simulink model "Traj_track_Mechanum_robot_Exp"  (R2024b)
settings: Solver=ode4  StartTime=0.0  StopTime=100  FixedStep=0.02  RelTol=1e-3  EnableMultiTasking=on
libraries: arduinolib x20, slpidlib x8
settings Model: ExtModeTrigDuration=2  Creator=my  LastModifiedBy=my
settings SolverCC: AutoInsertRateTranBlk=on
settings DataIOCC: SaveOutput=off  SignalLogging=off  DSMLogging=off  SaveTime=off  ReturnWorkspaceOutputs=off
settings OptimizationCC: EnhancedBackFolding=on  PassReuseOutputArgsAs=Individual arguments  ZeroExternalMemoryAtStartup=off  ZeroInternalMemoryAtStartup=off  MaxStackSize=64  OptimizeBlockOrder=speed  DifferentSizesBufferReuse=on  OptimizationCustomize=off  EfficientTunableParamExpr=on
settings DebuggingCC: ParameterTunabilityLossMsg=error
settings HardwareCC: ProdBitPerInt=16  ProdBitPerPointer=16  ProdBitPerSizeT=16  ProdBitPerPtrDiffT=16  ProdLargestAtomicFloat=None  ProdWordSize=8  ProdHWDeviceType=Atmel->AVR  UseEmbeddedCoderFeatures=off  UseSimulinkCoderFeatures=off
settings SFSimCC: MATLABDynamicMemAlloc=off
settings RTWCC: Description=Embedded Coder  SystemTargetFile=ert.tlc  HardwareBoard=Arduino Mega 2560  TemplateMakefile=ert_default_tmf  Toolchain=Arduino AVR  BuildConfiguration=Faster Runs
settings CodeAppCC: ForceParamTrailComments=on  IgnoreCustomStorageClasses=off  OperatorAnnotations=on  SimulinkDataObjDesc=on  SFDataObjDesc=on  MangleLength=10  InsertBlockDesc=on
settings ERTTargetCC: SupportContinuousTime=on  SupportNonInlinedSFcns=on  SupportVariableSizeSignals=on  ExtModeTransport=3  ExtModeStaticAlloc=on  ExtModeAutomaticAllocSize=off  ExtModeStaticAllocSize=2048  ExtModeMexFile=ext_xcp  ExtModeIntrfLevel=Level2 - Open  InlinedParameterPlacement=Hierarchical

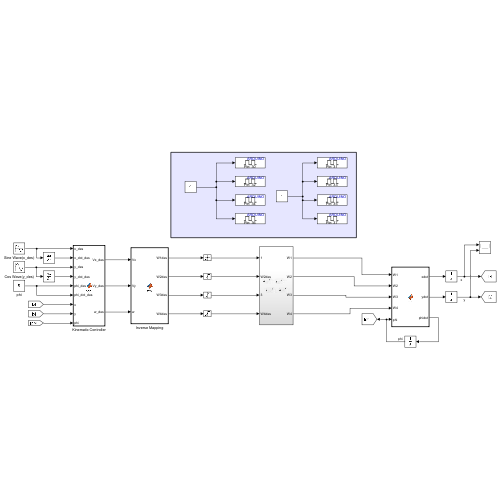
[thumbnail: Simulink's stored preview of the top-level diagram]
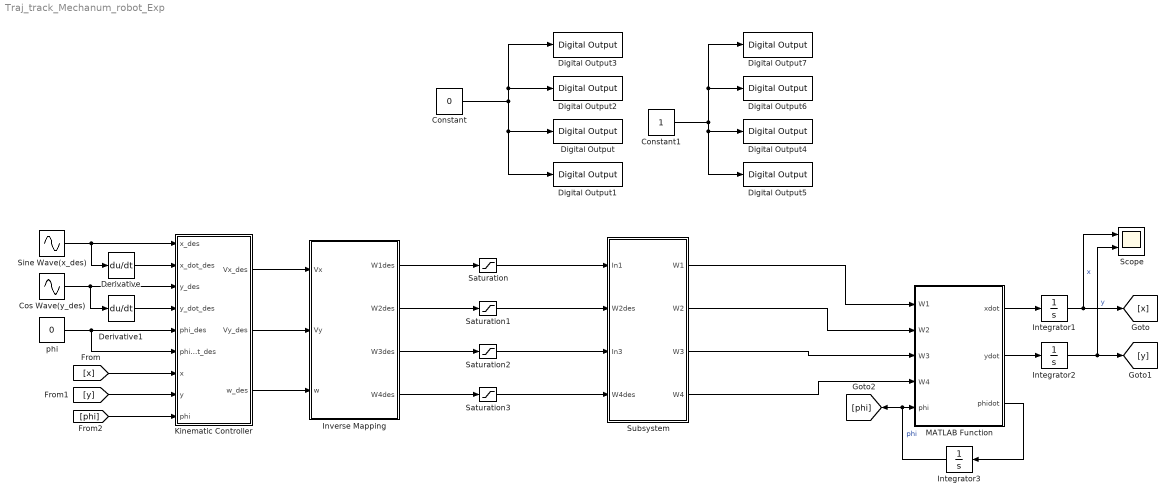
== system Traj_track_Mechanum_robot_Exp ==
  Constant : Constant  Value=0
  Constant1 : Constant
  Cos Wave(y_des) : Sin  Frequency=0.1  Phase=pi/2  SampleTime=0
  Derivative : Derivative
  Derivative1 : Derivative
  Digital Output : arduinolib/Digital Output  pinNumber=34  Direction=output  blockPlatform=arduino
  Digital Output1 : arduinolib/Digital Output  pinNumber=36  Direction=output  blockPlatform=arduino
  Digital Output2 : arduinolib/Digital Output  pinNumber=32  Direction=output  blockPlatform=arduino
  Digital Output3 : arduinolib/Digital Output  pinNumber=30  Direction=output  blockPlatform=arduino
  Digital Output4 : arduinolib/Digital Output  pinNumber=35  Direction=output  blockPlatform=arduino
  Digital Output5 : arduinolib/Digital Output  pinNumber=37  Direction=output  blockPlatform=arduino
  Digital Output6 : arduinolib/Digital Output  pinNumber=33  Direction=output  blockPlatform=arduino
  Digital Output7 : arduinolib/Digital Output  pinNumber=31  Direction=output  blockPlatform=arduino
  Integrator1 : Integrator
  Integrator2 : Integrator
  Integrator3 : Integrator
  Inverse Mapping : MATLAB Function  TreatAsAtomicUnit=on
  Kinematic Controller : MATLAB Function  TreatAsAtomicUnit=on
  MATLAB Function : MATLAB Function  TreatAsAtomicUnit=on
  Saturation : Saturate  UpperLimit=300  LowerLimit=-300
  Saturation1 : Saturate  UpperLimit=117  LowerLimit=-117
  Saturation2 : Saturate  UpperLimit=117  LowerLimit=-117
  Saturation3 : Saturate  UpperLimit=117  LowerLimit=-117
  Scope : Scope  NumInputPorts=2
  Sine Wave(x_des) : Sin  Frequency=0.1  SampleTime=0
  Subsystem : Subsystem
  phi : Constant  Value=0
  wires:
  Constant/1 -> Digital Output1/1, Digital Output/1, Digital Output2/1, Digital Output3/1
  Constant1/1 -> Digital Output6/1, Digital Output7/1, Digital Output5/1, Digital Output4/1
  Integrator2/1 -> Scope/2, [y]  "y"
  MATLAB Function/2(ydot) -> Integrator2/1
  MATLAB Function/1(xdot) -> Integrator1/1
  Integrator3/1 -> [phi], MATLAB Function/5(phi)  "phi"
  MATLAB Function/3(phidot) -> Integrator3/1
  Integrator1/1 -> Scope/1, [x]  "x"
  Saturation/1 -> Subsystem/1(In1)
  Saturation1/1 -> Subsystem/2(W2des)
  Saturation2/1 -> Subsystem/3(In3)
  Saturation3/1 -> Subsystem/4(W4des)
  Subsystem/1(W1) -> MATLAB Function/1(W1)
  Subsystem/2(W2) -> MATLAB Function/2(W2)
  Subsystem/3(W3) -> MATLAB Function/3(W3)
  Subsystem/4(W4) -> MATLAB Function/4(W4)
  Cos Wave(y_des)/1 -> Derivative1/1, Kinematic Controller/3(y_des)
  [phi] -> Kinematic Controller/9(phi)
  Inverse Mapping/1(W1des) -> Saturation/1
  Inverse Mapping/4(W4des) -> Saturation3/1
  [x] -> Kinematic Controller/7(x)
  Derivative/1 -> Kinematic Controller/2(x_dot_des)
  Kinematic Controller/1(Vx_des) -> Inverse Mapping/1(Vx)
  Kinematic Controller/2(Vy_des) -> Inverse Mapping/2(Vy)
  Inverse Mapping/3(W3des) -> Saturation2/1
  Kinematic Controller/3(w_des) -> Inverse Mapping/3(w)
  [y] -> Kinematic Controller/8(y)
  Inverse Mapping/2(W2des) -> Saturation1/1
  Sine Wave(x_des)/1 -> Derivative/1, Kinematic Controller/1(x_des)
  Derivative1/1 -> Kinematic Controller/4(y_dot_des)
  phi/1 -> Kinematic Controller/6(phi_dot_des), Kinematic Controller/5(phi_des)

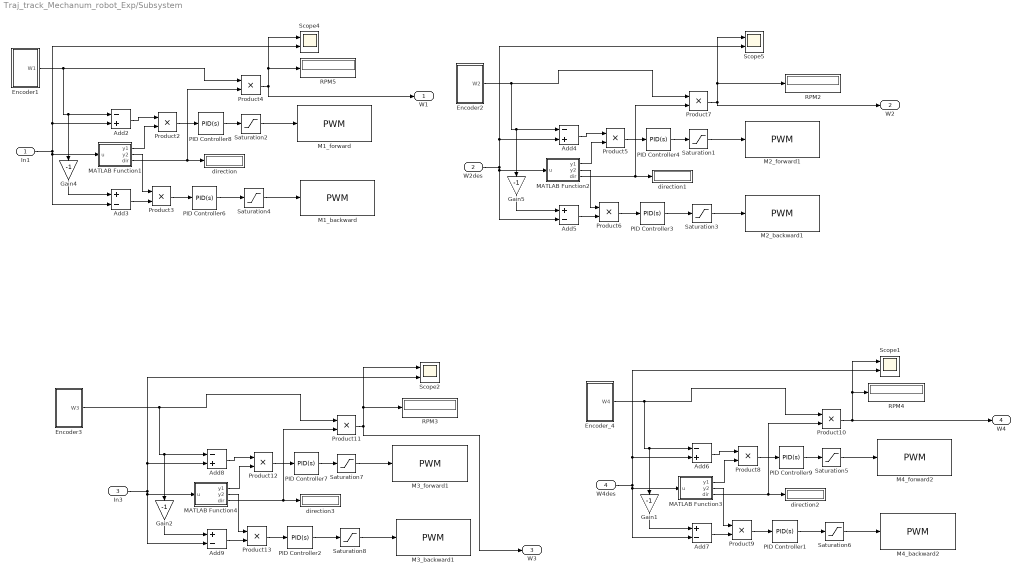
== system Traj_track_Mechanum_robot_Exp/Subsystem ==
  In1 : Inport
  W2des : Inport  Port=2
  In3 : Inport  Port=3
  W4des : Inport  Port=4
  Add{2,4,6,8} (4 alike) : Sum  Inputs=-+
  Add{3,5,7,9} (4 alike) : Sum  Inputs=+-
  Encoder1 : Subsystem
  Encoder2 : Subsystem
  Encoder3 : Subsystem
  Encoder_4 : Subsystem
  Gain{1..2,4..5} (4 alike) : Gain  Gain=-1
  M1_backward : arduinolib/PWM  pinNumber=5  frequencyType=Default  desiredFrequency=490.2  achievableFrequency=490.2
  M1_forward : arduinolib/PWM  pinNumber=4  frequencyType=Default  desiredFrequency=490.2  achievableFrequency=490.2
  M2_backward1 : arduinolib/PWM  pinNumber=7  frequencyType=Default  desiredFrequency=490.2  achievableFrequency=490.2
  M2_forward1 : arduinolib/PWM  pinNumber=6  frequencyType=Default  desiredFrequency=490.2  achievableFrequency=490.2
  M3_backward1 : arduinolib/PWM  pinNumber=10  frequencyType=Default  desiredFrequency=490.2  achievableFrequency=490.2
  M3_forward1 : arduinolib/PWM  pinNumber=9  frequencyType=Default  desiredFrequency=490.2  achievableFrequency=490.2
  M4_backward2 : arduinolib/PWM  pinNumber=12  frequencyType=Default  desiredFrequency=490.2  achievableFrequency=490.2
  M4_forward2 : arduinolib/PWM  pinNumber=11  frequencyType=Default  desiredFrequency=490.2  achievableFrequency=490.2
  MATLAB Function1 : MATLAB Function  TreatAsAtomicUnit=on
  MATLAB Function2 : MATLAB Function  TreatAsAtomicUnit=on
  MATLAB Function3 : MATLAB Function  TreatAsAtomicUnit=on
  MATLAB Function4 : MATLAB Function  TreatAsAtomicUnit=on
  PID Controller{1..4,6..9} (8 alike) : slpidlib/PID Controller  Controller=PID  Form=Parallel  TimeDomain=Continuous-time  UseExternalTs=off  SampleTime=-1  IntegratorMethod=Forward Euler  FilterMethod=Forward Euler  ControllerParametersSource=internal  P=10  I=0  UseKiTs=off  D=0  UseExternalDerivativeSource=off  N=100  UseFilter=on  TunerSelectOption=Transfer Function Based (PID Tuner App)  InitialConditionSource=internal  InitialConditionForIntegrator=0  InitialConditionForFilter=0  DifferentiatorICPrevScaledInput=0  ExternalReset=none  TrackingMode=off  Kt=1  LimitOutput=on  SatLimitsSource=internal  UpperSaturationLimit=255  LowerSaturationLimit=0  LinearizeAsGain=on  AntiWindupMode=none  Kb=1  LimitIntegrator=off  UpperIntegratorSaturationLimit=inf  LowerIntegratorSaturationLimit=-inf  POutMin=[]  POutMax=[]  IOutMin=[]  IOutMax=[]  DOutMin=[]  DOutMax=[]  NOutMin=[]  NOutMax=[]  SumOutMin=[]  SumOutMax=[]  SaturationOutMin=[]  SaturationOutMax=[]  PParamMin=[]  PParamMax=[]  IParamMin=[]  IParamMax=[]  DParamMin=[]  DParamMax=[]  NParamMin=[]  NParamMax=[]  KbParamMin=[]  KbParamMax=[]  KtParamMin=[]  KtParamMax=[]  KbOutMin=[]  KbOutMax=[]  KtOutMin=[]  KtOutMax=[]  IntegratorOutMin=[]  IntegratorOutMax=[]  FilterOutMin=[]  FilterOutMax=[]  SumI1OutMin=[]  SumI1OutMax=[]  SumI2OutMin=[]  SumI2OutMax=[]  SumI3OutMin=[]  SumI3OutMax=[]  SumI4OutMin=[]  SumI4OutMax=[]  SumDOutMin=[]  SumDOutMax=[]  DifferentiatorOutMin=[]  DifferentiatorOutMax=[]  FilterDiffOutCoefMin=[]  FilterDiffOutCoefMax=[]  ReciprocalOutMin=[]  ReciprocalOutMax=[]  SumDenOutMin=[]  SumDenOutMax=[]  SumNumOutMin=[]  SumNumOutMax=[]  DivideOutMin=[]  DivideOutMax=[]  UdiffTsProdOutMin=[]  UdiffTsProdOutMax=[]  NTsProdOutMin=[]  NTsProdOutMax=[]  UintegralTsProdOutMin=[]  UintegralTsProdOutMax=[]  UngainTsProdOutMin=[]  UngainTsProdOutMax=[]  ClampingZeroOutDataTypeStr=Inherit: Inherit via back propagation  ClampingZeroOutMin=[]  ClampingZeroOutMax=[]  FilterDenConstantOutDataTypeStr=Inherit: Inherit via back propagation  FilterDenConstantOutMin=[]  FilterDenConstantOutMax=[]  PCopyOutDataTypeStr=Inherit: Inherit via back propagation  PCopyOutMin=[]  PCopyOutMax=[]  NCopyOutDataTypeStr=Inherit: Inherit via back propagation  NCopyOutMin=[]  NCopyOutMax=[]  IntegratorContinuousStateAttributes=''  IntegratorStateMustResolveToSignalObject=off  IntegratorRTWStateStorageClass=Auto  FilterContinuousStateAttributes=''  FilterStateMustResolveToSignalObject=off  FilterRTWStateStorageClass=Auto  ParallelPVariant=InternalParameters  IdealPVariant=Disabled  IVariant=InternalParameters  DVariant=InternalParameters  IntegratorVariant=Continuous  SatVariant=Enabled  AWVariant=Passthrough  PCopyVariant=Disabled  TRVariant=Disabled  FdbkBlocksVariant=Forward  IdealPFdbkVariant=Disabled  SatFdbkVariant=Disabled  DerivativeFilterVariant=ContFilter  NVariant=InternalParameters  NCopyVariant=Disabled  FilterICVariant=InternalICsFilter  IntegratorICVariant=InternalICs  ExternalResetVariant=Disabled  TRSumVariant=Passthrough  SumFdbkVariant=Disabled  SumVariant=Sum_PID  TsampFilterVariant=InternalTs  TsampNgainVariant=Passthrough  TsampIntegralVariant=Disabled_SignalSpec  ExternalSaturationOutDataTypeStr=Inherit: Same as second input  DerivativeSourceVariant=ErrorSignal  PreIntVariant=InternalPreInt
  Product{2..13} (12 alike) : Product
  RPM{2..5} (4 alike) : Display
  Saturation{1..8} (8 alike) : Saturate  UpperLimit=250  LowerLimit=0
  Scope{1..2,4..5} (4 alike) : Scope  NumInputPorts=2
  direction{,1..3} (4 alike) : Display
  W1 : Outport
  W2 : Outport  Port=2
  W3 : Outport  Port=3
  W4 : Outport  Port=4
  wires:
  MATLAB Function1/2(y2) -> Product3/1
  MATLAB Function1/3(dir) -> Product4/2, direction/1
  In1/1 -> Scope4/2, Add2/2, Add3/2, MATLAB Function1/1(u)
  PID Controller6/1 -> Saturation4/1
  Saturation2/1 -> M1_forward/1
  PID Controller8/1 -> Saturation2/1
  Saturation4/1 -> M1_backward/1
  Add2/1 -> Product2/1
  Encoder1/1(W1) -> Product4/1, Add2/1, Gain4/1
  MATLAB Function1/1(y1) -> Product2/2
  Product2/1 -> PID Controller8/1
  Gain4/1 -> Add3/1
  Product3/1 -> PID Controller6/1
  Add3/1 -> Product3/2
  Add5/1 -> Product6/2
  Product6/1 -> PID Controller3/1
  Gain5/1 -> Add5/1
  Product5/1 -> PID Controller4/1
  MATLAB Function2/1(y1) -> Product5/2
  Encoder2/1(W2) -> Gain5/1, Add4/1, Product7/1
  Add4/1 -> Product5/1
  Saturation3/1 -> M2_backward1/1
  PID Controller4/1 -> Saturation1/1
  Saturation1/1 -> M2_forward1/1
  PID Controller3/1 -> Saturation3/1
  W2des/1 -> MATLAB Function2/1(u), Add5/2, Add4/2, Scope5/2
  MATLAB Function2/3(dir) -> direction1/1, Product7/2
  MATLAB Function2/2(y2) -> Product6/1
  MATLAB Function3/2(y2) -> Product9/1
  MATLAB Function3/3(dir) -> Product10/2, direction2/1
  W4des/1 -> Scope1/2, Add6/2, Add7/2, MATLAB Function3/1(u)
  PID Controller1/1 -> Saturation6/1
  Saturation5/1 -> M4_forward2/1
  PID Controller9/1 -> Saturation5/1
  Saturation6/1 -> M4_backward2/1
  Add6/1 -> Product8/1
  Encoder_4/1(W4) -> Product10/1, Add6/1, Gain1/1
  MATLAB Function3/1(y1) -> Product8/2
  Product8/1 -> PID Controller9/1
  Gain1/1 -> Add7/1
  Product9/1 -> PID Controller1/1
  Add7/1 -> Product9/2
  Product11/1 -> Scope2/1, RPM3/1, W3/1
  Add9/1 -> Product13/2
  Product13/1 -> PID Controller2/1
  Gain2/1 -> Add9/1
  Product12/1 -> PID Controller7/1
  MATLAB Function4/1(y1) -> Product12/2
  Encoder3/1(W3) -> Gain2/1, Add8/1, Product11/1
  Add8/1 -> Product12/1
  Saturation8/1 -> M3_backward1/1
  PID Controller7/1 -> Saturation7/1
  PID Controller2/1 -> Saturation8/1
  In3/1 -> MATLAB Function4/1(u), Add9/2, Add8/2, Scope2/2
  MATLAB Function4/3(dir) -> direction3/1, Product11/2
  MATLAB Function4/2(y2) -> Product13/1
  Saturation7/1 -> M3_forward1/1
  Product10/1 -> RPM4/1, Scope1/1, W4/1
  Product7/1 -> RPM2/1, Scope5/1, W2/1
  Product4/1 -> RPM5/1, Scope4/1, W1/1

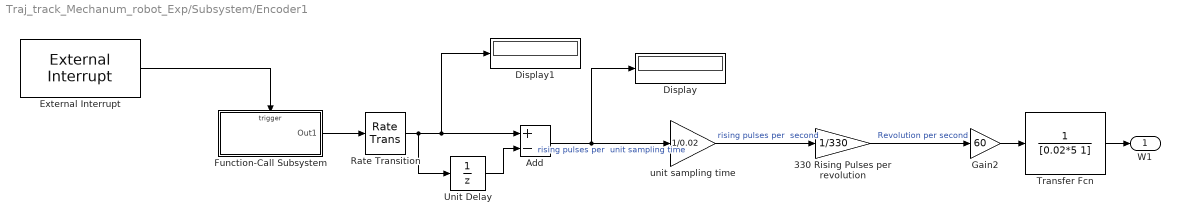
== system Traj_track_Mechanum_robot_Exp/Subsystem/Encoder1 ==
  330 Rising Pulses per revolution : Gain  Gain=1/330
  Add : Sum  Inputs=+-
  Display : Display
  Display1 : Display
  External Interrupt : arduinolib/External Interrupt  Pin=21  PullUp=off  Mode=RISING  InterruptSimulationInput=off
  Function-Call Subsystem : Subsystem  TreatAsAtomicUnit=on
  Gain2 : Gain  Gain=60
  Rate Transition : RateTransition  Integrity=off  Deterministic=off  OutPortSampleTimeOpt=Inherit
  Transfer Fcn : TransferFcn  Denominator=[0.02*5 1]
  Unit Delay : UnitDelay  SampleTime=0.02  HasFrameUpgradeWarning=on
  unit sampling time : Gain  Gain=1/0.02
  W1 : Outport
  wires:
  Transfer Fcn/1 -> W1/1
  Add/1 -> unit sampling time/1, Display/1  "rising pulses per  unit sampling time"
  External Interrupt/1 -> Function-Call Subsystem/Trigger
  Function-Call Subsystem/1(Out1) -> Rate Transition/1
  Gain2/1 -> Transfer Fcn/1
  330 Rising Pulses per revolution/1 -> Gain2/1  "Revolution per second"
  Rate Transition/1 -> Add/1, Display1/1, Unit Delay/1
  unit sampling time/1 -> 330 Rising Pulses per revolution/1  "rising pulses per  second"
  Unit Delay/1 -> Add/2

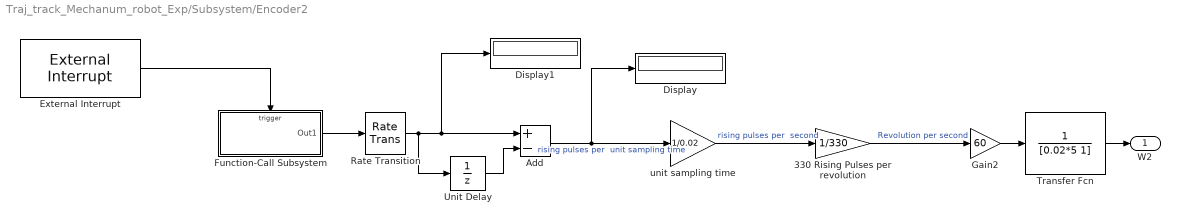
== system Traj_track_Mechanum_robot_Exp/Subsystem/Encoder2 ==
  330 Rising Pulses per revolution : Gain  Gain=1/330
  Add : Sum  Inputs=+-
  Display : Display
  Display1 : Display
  External Interrupt : arduinolib/External Interrupt  Pin=20  PullUp=off  Mode=RISING  InterruptSimulationInput=off
  Function-Call Subsystem : Subsystem  TreatAsAtomicUnit=on
  Gain2 : Gain  Gain=60
  Rate Transition : RateTransition  Integrity=off  Deterministic=off  OutPortSampleTimeOpt=Inherit
  Transfer Fcn : TransferFcn  Denominator=[0.02*5 1]
  Unit Delay : UnitDelay  SampleTime=0.02  HasFrameUpgradeWarning=on
  unit sampling time : Gain  Gain=1/0.02
  W2 : Outport
  wires:
  Unit Delay/1 -> Add/2
  unit sampling time/1 -> 330 Rising Pulses per revolution/1  "rising pulses per  second"
  Rate Transition/1 -> Unit Delay/1, Display1/1, Add/1
  330 Rising Pulses per revolution/1 -> Gain2/1  "Revolution per second"
  Gain2/1 -> Transfer Fcn/1
  Function-Call Subsystem/1(Out1) -> Rate Transition/1
  External Interrupt/1 -> Function-Call Subsystem/Trigger
  Add/1 -> Display/1, unit sampling time/1  "rising pulses per  unit sampling time"
  Transfer Fcn/1 -> W2/1

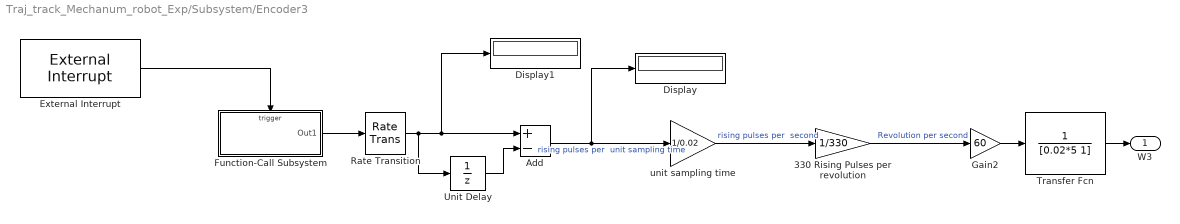
== system Traj_track_Mechanum_robot_Exp/Subsystem/Encoder3 ==
  330 Rising Pulses per revolution : Gain  Gain=1/330
  Add : Sum  Inputs=+-
  Display : Display
  Display1 : Display
  External Interrupt : arduinolib/External Interrupt  Pin=19  PullUp=off  Mode=RISING  InterruptSimulationInput=off
  Function-Call Subsystem : Subsystem  TreatAsAtomicUnit=on
  Gain2 : Gain  Gain=60
  Rate Transition : RateTransition  Integrity=off  Deterministic=off  OutPortSampleTimeOpt=Inherit
  Transfer Fcn : TransferFcn  Denominator=[0.02*5 1]
  Unit Delay : UnitDelay  SampleTime=0.02  HasFrameUpgradeWarning=on
  unit sampling time : Gain  Gain=1/0.02
  W3 : Outport
  wires:
  Transfer Fcn/1 -> W3/1
  Add/1 -> unit sampling time/1, Display/1  "rising pulses per  unit sampling time"
  External Interrupt/1 -> Function-Call Subsystem/Trigger
  Function-Call Subsystem/1(Out1) -> Rate Transition/1
  Gain2/1 -> Transfer Fcn/1
  330 Rising Pulses per revolution/1 -> Gain2/1  "Revolution per second"
  Rate Transition/1 -> Add/1, Display1/1, Unit Delay/1
  unit sampling time/1 -> 330 Rising Pulses per revolution/1  "rising pulses per  second"
  Unit Delay/1 -> Add/2

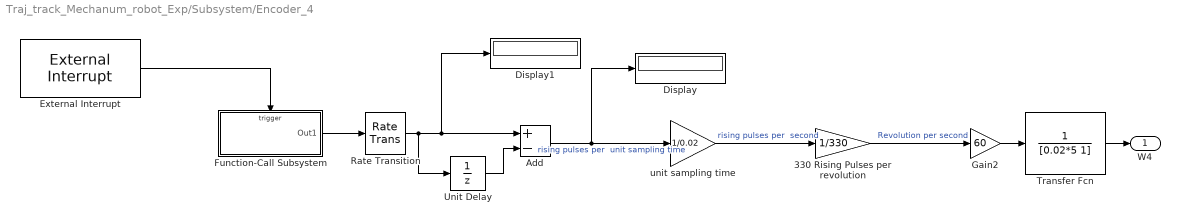
== system Traj_track_Mechanum_robot_Exp/Subsystem/Encoder_4 ==
  330 Rising Pulses per revolution : Gain  Gain=1/330
  Add : Sum  Inputs=+-
  Display : Display
  Display1 : Display
  External Interrupt : arduinolib/External Interrupt  Pin=18  PullUp=off  Mode=RISING  InterruptSimulationInput=off
  Function-Call Subsystem : Subsystem  TreatAsAtomicUnit=on
  Gain2 : Gain  Gain=60
  Rate Transition : RateTransition  Integrity=off  Deterministic=off  OutPortSampleTimeOpt=Inherit
  Transfer Fcn : TransferFcn  Denominator=[0.02*5 1]
  Unit Delay : UnitDelay  SampleTime=0.02  HasFrameUpgradeWarning=on
  unit sampling time : Gain  Gain=1/0.02
  W4 : Outport
  wires:
  Unit Delay/1 -> Add/2
  unit sampling time/1 -> 330 Rising Pulses per revolution/1  "rising pulses per  second"
  Rate Transition/1 -> Unit Delay/1, Display1/1, Add/1
  330 Rising Pulses per revolution/1 -> Gain2/1  "Revolution per second"
  Gain2/1 -> Transfer Fcn/1
  Function-Call Subsystem/1(Out1) -> Rate Transition/1
  External Interrupt/1 -> Function-Call Subsystem/Trigger
  Add/1 -> Display/1, unit sampling time/1  "rising pulses per  unit sampling time"
  Transfer Fcn/1 -> W4/1

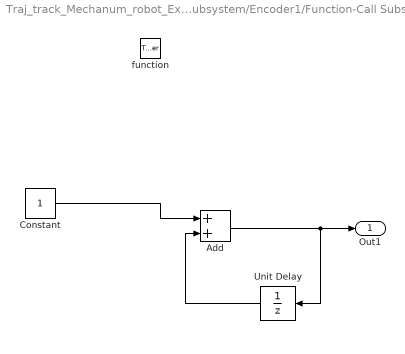
== system Traj_track_Mechanum_robot_Exp/Subsystem/Encoder1/Function-Call Subsystem ==
  function : TriggerPort  TriggerType=function-call  VariantControl=(inherit)
  Add : Sum
  Constant : Constant
  Unit Delay : UnitDelay  SampleTime=-1  HasFrameUpgradeWarning=on
  Out1 : Outport
  wires:
  Constant/1 -> Add/1
  Unit Delay/1 -> Add/2
  Add/1 -> Out1/1, Unit Delay/1

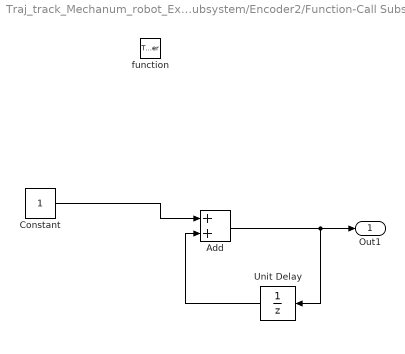
== system Traj_track_Mechanum_robot_Exp/Subsystem/Encoder2/Function-Call Subsystem ==
  function : TriggerPort  TriggerType=function-call  VariantControl=(inherit)
  Add : Sum
  Constant : Constant
  Unit Delay : UnitDelay  SampleTime=-1  HasFrameUpgradeWarning=on
  Out1 : Outport
  wires:
  Add/1 -> Unit Delay/1, Out1/1
  Unit Delay/1 -> Add/2
  Constant/1 -> Add/1

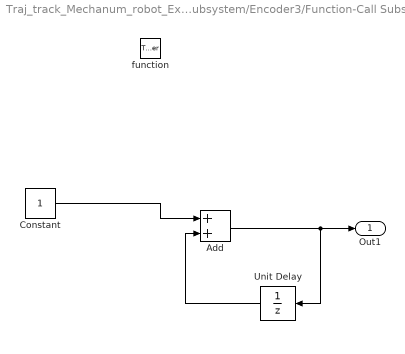
== system Traj_track_Mechanum_robot_Exp/Subsystem/Encoder3/Function-Call Subsystem ==
  function : TriggerPort  TriggerType=function-call  VariantControl=(inherit)
  Add : Sum
  Constant : Constant
  Unit Delay : UnitDelay  SampleTime=-1  HasFrameUpgradeWarning=on
  Out1 : Outport
  wires:
  Constant/1 -> Add/1
  Unit Delay/1 -> Add/2
  Add/1 -> Out1/1, Unit Delay/1

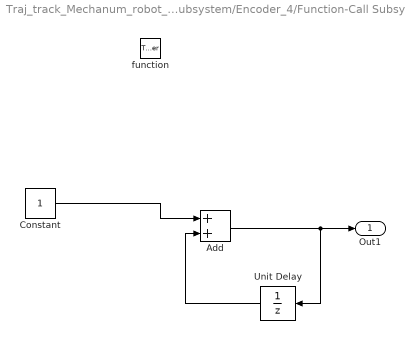
== system Traj_track_Mechanum_robot_Exp/Subsystem/Encoder_4/Function-Call Subsystem ==
  function : TriggerPort  TriggerType=function-call  VariantControl=(inherit)
  Add : Sum
  Constant : Constant
  Unit Delay : UnitDelay  SampleTime=-1  HasFrameUpgradeWarning=on
  Out1 : Outport
  wires:
  Add/1 -> Unit Delay/1, Out1/1
  Unit Delay/1 -> Add/2
  Constant/1 -> Add/1

== matlab function Traj_track_Mechanum_robot_Exp/Inverse Mapping ==
  data: Vx input; W1des output; W2des output; W3des output; W4des output; Vy input; w input
function [W1des,W2des,W3des,W4des] = fcn(Vx,Vy,w)

r = 0.04;
Lx = 0.09;
Ly = 0.095;
%% Define matrix M

M = (1/r)*[1,-1,-(Lx+Ly); 1,1,(Lx+Ly); 1,1,-(Lx+Ly); 1,-1,(Lx+Ly)];

Wheel_speeds = M*[Vx;Vy;w];

W1des = Wheel_speeds(1);
W2des =  Wheel_speeds(2);
W3des = Wheel_speeds(3);
W4des =  Wheel_speeds(4);

%convert rad/sec to RPM

W1des = (60/(2*pi))*W1des;
W2des = (60/(2*pi))*W2des;
W3des = (60/(2*pi))*W3des;
W4des = (60/(2*pi))*W4des;

%%

== matlab function Traj_track_Mechanum_robot_Exp/MATLAB Function ==
  data: W1 input; xdot output; W2 input; W3 input; W4 input; ydot output; phidot output; phi input
function [xdot,ydot,phidot] = fcn(W1,W2,W3,W4,phi)

r = 0.04;
Lx = 0.09;
Ly = 0.095;

%convert RW,LW from RPM to rad/sec.

W1 = W1*(2*pi/60);
W2 = W2*(2*pi/60);
W3 = W3*(2*pi/60);
W4 = W4*(2*pi/60);

Vx = r*(W1 + W2 + W3 + W4)/4;
Vy = r*(-W1 + W2 + W3 - W4)/4;
w = r*(-W1 + W2 -W3 + W4)/(4*(Lx+Ly));


xdot = Vx*cos(phi) - Vy*sin(phi);
ydot = Vy*sin(phi) + Vy*cos(phi);
phidot = w;

== matlab function Traj_track_Mechanum_robot_Exp/Kinematic Controller ==
  data: x_des input; x_dot_des input; Vx_des output; y_des input; y_dot_des input; phi_des input; phi_dot_des input; x input; y input; Vy_des output; w_des output; phi input
function [Vx_des,Vy_des,w_des] = fcn(x_des,x_dot_des,y_des,y_dot_des,phi_des, phi_dot_des, x,y,phi)

T = [cos(phi),-sin(phi),0;
     sin(phi),cos(phi),0;
     0,0,1];

kx = 3;
ky = 3;
kphi = 1;

V = inv(T)*[x_dot_des + kx* tanh(x_des - x);
            y_dot_des + ky* tanh(y_des - y);
            phi_dot_des + kphi* tanh(phi_des - phi)];

Vx_des = V(1);
Vy_des = V(2);
w_des = V(3);

== matlab function Traj_track_Mechanum_robot_Exp/Subsystem/MATLAB Function1 ==
  data: u input; y1 output; y2 output; dir output
function [y1,y2,dir] = fcn(u)

if u > 0 
    y1 = 1;
    y2 = 0;
    dir = 1;
else
    y1 = 0;
    y2 = 1;
    dir = -1;
end

== matlab function Traj_track_Mechanum_robot_Exp/Subsystem/MATLAB Function2 ==
  data: u input; y1 output; y2 output; dir output
function [y1,y2,dir] = fcn(u)

if u > 0 
    y1 = 1;
    y2 = 0;
    dir = 1;
else
    y1 = 0;
    y2 = 1;
    dir = -1;
end

== matlab function Traj_track_Mechanum_robot_Exp/Subsystem/MATLAB Function3 ==
  data: u input; y1 output; y2 output; dir output
function [y1,y2,dir] = fcn(u)

if u > 0 
    y1 = 1;
    y2 = 0;
    dir = 1;
else
    y1 = 0;
    y2 = 1;
    dir = -1;
end

== matlab function Traj_track_Mechanum_robot_Exp/Subsystem/MATLAB Function4 ==
  data: u input; y1 output; y2 output; dir output
function [y1,y2,dir] = fcn(u)

if u > 0 
    y1 = 1;
    y2 = 0;
    dir = 1;
else
    y1 = 0;
    y2 = 1;
    dir = -1;
end
